simulink model "FullCarModel"  (R2023a)
settings: Solver=FixedStepAuto  StartTime=0.0  StopTime=10.0  FixedStep=5e-3  RelTol=1e-3
values from neighbouring files (symbols this model uses):
  z_r_type = 1    [FullCarParameters.m]
undefined symbols (not defined in the file or in its folder): a1F, a2F, aero, BF, CF, chassis, constants, EF, suspension
libraries: simulink x3
settings Model: Creator=Cassio de Freitas  LastModifiedBy=Cassio de Freitas
settings DataIOCC: ReturnWorkspaceOutputsName=simout

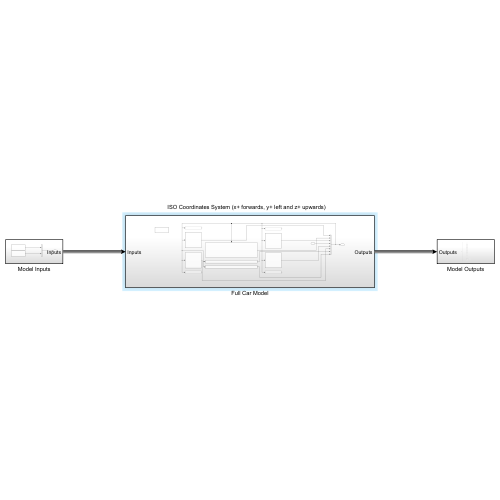
[thumbnail: Simulink's stored preview of the top-level diagram]
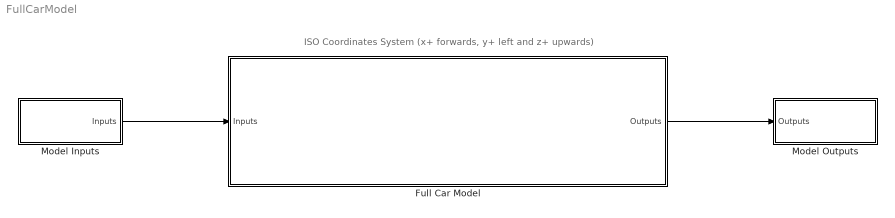
== system FullCarModel ==
  note: ISO Coordinates System (x+ forwards, y+ left and z+ upwards)
  Full Car Model : Subsystem
  Model Inputs : Subsystem
  Model Outputs : Subsystem
  wires:
  Full Car Model/1(Outputs) -> Model Outputs/1(Outputs)
  Model Inputs/1(Inputs) -> Full Car Model/1(Inputs)

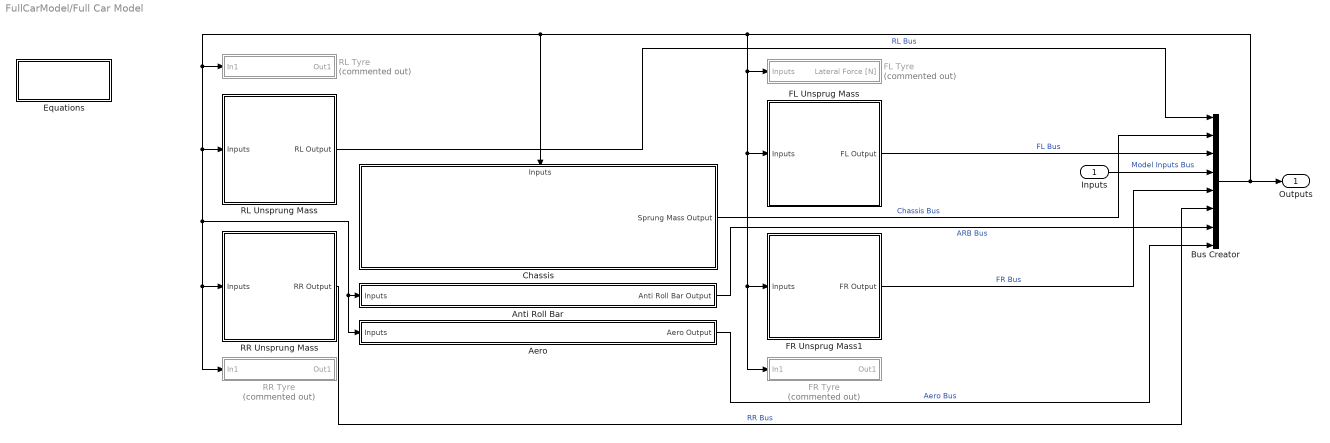
== system FullCarModel/Full Car Model ==
  Inputs : Inport
  Aero : Subsystem
  Anti Roll Bar : Subsystem
  Bus Creator : BusCreator  Inputs=8
  Chassis : Subsystem
      settings: PortSchema="{\"entries\":[{\"content\":{\"sides\":[{\"content\":{},\"type\":\"ConnectorPlacement.EquallySpacedRectSide\",\"uuid\":\"63b5c35c-1345-4ade-85d7-a7aac4cc3700\"},{\"content\":{\"connectorIds\":[\"Out1\"],\"side\":\"RIGHT\"},\"type\":\"ConnectorPlacement.EquallySpacedRectSide\",\"uuid\":\"42c6bf5f-ecea-40ec-868a-6613098306c6\"},{\"content\":{\"connectorIds\":[\"In1\"],\"side\":\"TOP\"},\"type\":\"ConnectorPlacement.EquallySpacedRectSide\",\"uuid\":\"4661345b-8a90-4c28-8ce6-d1521a801330\"}]},\"type\":\"ConnectorPlacement.EquallySpacedConnector\",\"uuid\":\"31a4e6e8-77fc-45d3-842e-fbcb04573c93\"}],\"packageUris\":[\"http://schema.mathworks.com/mf0/Connector/R2020b\"],\"version\":\"1.0\"}"
  Equations : Subsystem
  FL Tyre : Subsystem  Commented=on
  FL Unsprug Mass : Subsystem
  FR Tyre : Subsystem  Commented=on
  FR Unsprug Mass1 : Subsystem
  RL Tyre : Subsystem  Commented=on
  RL Unsprung Mass : Subsystem
  RR Tyre : Subsystem  Commented=on
  RR Unsprung Mass : Subsystem
  Outputs : Outport
  wires:
  RL Unsprung Mass/1(RL Output) -> Bus Creator/1  "RL Bus"
  Chassis/1(Sprung Mass Output) -> Bus Creator/2  "Chassis Bus"
  FL Unsprug Mass/1(FL Output) -> Bus Creator/3  "FL Bus"
  Bus Creator/1 -> Chassis/1(Inputs), RL Tyre/1(In1), RL Unsprung Mass/1(Inputs), RR Unsprung Mass/1(Inputs), RR Tyre/1(In1), Aero/1(Inputs), Anti Roll Bar/1(Inputs), FL Tyre/1(Inputs), FL Unsprug Mass/1(Inputs), FR Unsprug Mass1/1(Inputs), FR Tyre/1(In1), Outputs/1
  Inputs/1 -> Bus Creator/4  "Model Inputs Bus"
  FR Unsprug Mass1/1(FR Output) -> Bus Creator/5  "FR Bus"
  RR Unsprung Mass/1(RR Output) -> Bus Creator/6  "RR Bus"
  Anti Roll Bar/1(Anti Roll Bar Output) -> Bus Creator/7  "ARB Bus"
  Aero/1(Aero Output) -> Bus Creator/8  "Aero Bus"

== system FullCarModel/Model Inputs ==
  Driver Inputs : Subsystem
  Model Inputs Bus : BusCreator  Inputs=2
  Subsystem : Subsystem
  Inputs : Outport
  wires:
  Subsystem/1(Surface Model) -> Model Inputs Bus/1  "Surface Inputs"
  Model Inputs Bus/1 -> Inputs/1
  Driver Inputs/1(Driver Model) -> Model Inputs Bus/2  "Driver Inputs"

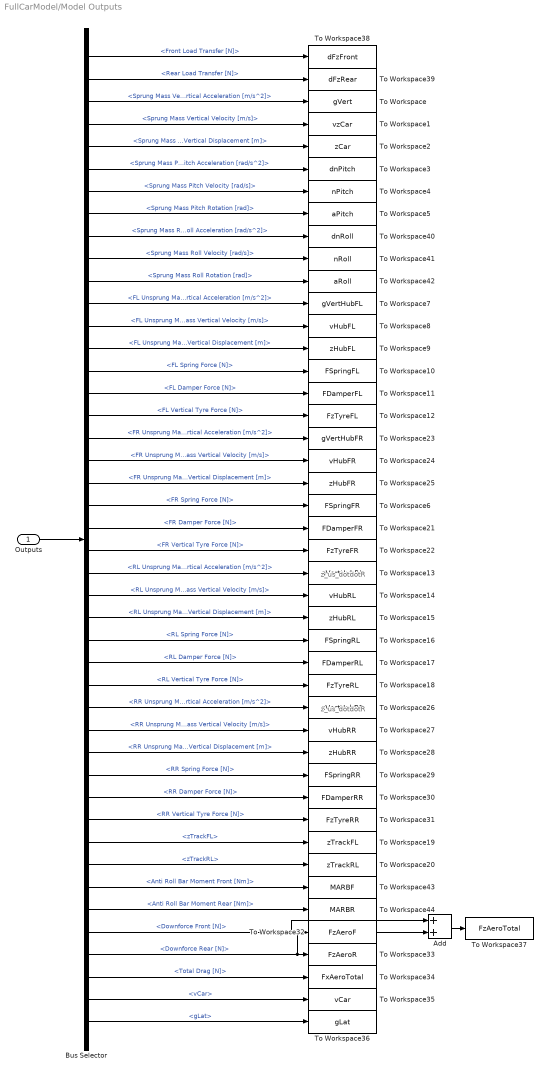
== system FullCarModel/Model Outputs ==
  note: z_us_dotdotR
  note: z_us_dotdotR
  Outputs : Inport
  Add : Sum
  Bus Selector : BusSelector  OutputSignals=FL Bus.Front Load Transfer [N],RL Bus.Rear Load Transfer [N],Chassis Bus.Sprung Mass Vertical Acceleration [m/s^2],Chassis Bus.Sprung Mass Vertical Velocity [m/s],Chassis Bus.Sprung Mass Vertical Displacement [m],Chassis Bus.Sprung Mass Pitch Acceleration [rad/s^2],Chassis Bus.Sprung Mass Pitch Velocity [rad/s],Chassis Bus.Sprung Mass Pitch Rotation [rad],Chassis Bus.Sprung Mass Roll Acceleration [rad/s^2],Chassis Bus.Sprung Mass Roll Velocity [rad/s],Chassis Bus.Sprung Mass Roll Rotation [rad],FL Bus.FL Unsprung Mass Vertical Acceleration [m/s^2],FL Bus.FL Unsprung Mass Vertical Velocity [m/s],FL Bus.FL Unsprung Mass Vertical Displacement [m],FL Bus.FL Spring Force [N],FL Bus.FL Damper Force [N],FL Bus.FL Vertical Tyre Force [N],FR Bus.FR Unsprung Mass Vertical Acceleration [m/s^2],FR Bus.FR Unsprung Mass Vertical Velocity [m/s],FR Bus.FR Unsprung Mass Vertical Displacement [m],FR Bus.FR Spring Force [N],FR Bus.FR Damper Force [N],FR Bus.FR Vertical Tyre Force [N],RL Bus.RL Unsprung Mass Vertical Acceleration [m/s^2],RL Bus.RL Unsprung Mass Vertical Velocity [m/s],RL Bus.RL Unsprung Mass Vertical Displacement [m],RL Bus.RL Spring Force [N],RL Bus.RL Damper Force [N],RL Bus.RL Vertical Tyre Force [N],RR Bus.RR Unsprung Mass Vertical Acceleration [m/s^2],RR Bus.RR Unsprung Mass Vertical Velocity [m/s],RR Bus.RR Unsprung Mass Vertical Displacement [m],RR Bus.RR Spring Force [N],RR Bus.RR Damper Force [N],RR Bus.RR Vertical Tyre Force [N],Model Inputs Bus.Surface Inputs.zTrackFL,Model Inputs Bus.Surface Inputs.zTrackRL,ARB Bus.Anti Roll Bar Moment Front [Nm],ARB Bus.Anti Roll Bar Moment Rear [Nm],Aero Bus.Downforce Front [N],Aero Bus.Downforce Rear [N],Aero Bus.Total Drag [N],Model Inputs Bus.Driver Inputs.vCar,Model Inputs Bus.Driver Inputs.gLat
  To Workspace : ToWorkspace  VariableName=gVert  SaveFormat=Timeseries  SampleTime=-1
  To Workspace1 : ToWorkspace  VariableName=vzCar  SaveFormat=Timeseries  SampleTime=-1
  To Workspace10 : ToWorkspace  VariableName=FSpringFL  SaveFormat=Timeseries  SampleTime=-1
  To Workspace11 : ToWorkspace  VariableName=FDamperFL  SaveFormat=Timeseries  SampleTime=-1
  To Workspace12 : ToWorkspace  VariableName=FzTyreFL  SaveFormat=Timeseries  SampleTime=-1
  To Workspace13 : ToWorkspace  VariableName=gVertHubRL  SaveFormat=Timeseries  SampleTime=-1
  To Workspace14 : ToWorkspace  VariableName=vHubRL  SaveFormat=Timeseries  SampleTime=-1
  To Workspace15 : ToWorkspace  VariableName=zHubRL  SaveFormat=Timeseries  SampleTime=-1
  To Workspace16 : ToWorkspace  VariableName=FSpringRL  SaveFormat=Timeseries  SampleTime=-1
  To Workspace17 : ToWorkspace  VariableName=FDamperRL  SaveFormat=Timeseries  SampleTime=-1
  To Workspace18 : ToWorkspace  VariableName=FzTyreRL  SaveFormat=Timeseries  SampleTime=-1
  To Workspace19 : ToWorkspace  VariableName=zTrackFL  SaveFormat=Timeseries  SampleTime=-1
  To Workspace2 : ToWorkspace  VariableName=zCar  SaveFormat=Timeseries  SampleTime=-1
  To Workspace20 : ToWorkspace  VariableName=zTrackRL  SaveFormat=Timeseries  SampleTime=-1
  To Workspace21 : ToWorkspace  VariableName=FDamperFR  SaveFormat=Timeseries  SampleTime=-1
  To Workspace22 : ToWorkspace  VariableName=FzTyreFR  SaveFormat=Timeseries  SampleTime=-1
  To Workspace23 : ToWorkspace  VariableName=gVertHubFR  SaveFormat=Timeseries  SampleTime=-1
  To Workspace24 : ToWorkspace  VariableName=vHubFR  SaveFormat=Timeseries  SampleTime=-1
  To Workspace25 : ToWorkspace  VariableName=zHubFR  SaveFormat=Timeseries  SampleTime=-1
  To Workspace26 : ToWorkspace  VariableName=gVertHubRR  SaveFormat=Timeseries  SampleTime=-1
  To Workspace27 : ToWorkspace  VariableName=vHubRR  SaveFormat=Timeseries  SampleTime=-1
  To Workspace28 : ToWorkspace  VariableName=zHubRR  SaveFormat=Timeseries  SampleTime=-1
  To Workspace29 : ToWorkspace  VariableName=FSpringRR  SaveFormat=Timeseries  SampleTime=-1
  To Workspace3 : ToWorkspace  VariableName=dnPitch  SaveFormat=Timeseries  SampleTime=-1
  To Workspace30 : ToWorkspace  VariableName=FDamperRR  SaveFormat=Timeseries  SampleTime=-1
  To Workspace31 : ToWorkspace  VariableName=FzTyreRR  SaveFormat=Timeseries  SampleTime=-1
  To Workspace32 : ToWorkspace  VariableName=FzAeroF  SaveFormat=Timeseries  SampleTime=-1
  To Workspace33 : ToWorkspace  VariableName=FzAeroR  SaveFormat=Timeseries  SampleTime=-1
  To Workspace34 : ToWorkspace  VariableName=FxAeroTotal  SaveFormat=Timeseries  SampleTime=-1
  To Workspace35 : ToWorkspace  VariableName=vCar  SaveFormat=Timeseries  SampleTime=-1
  To Workspace36 : ToWorkspace  VariableName=gLat  SaveFormat=Timeseries  SampleTime=-1
  To Workspace37 : ToWorkspace  VariableName=FzAeroTotal  SaveFormat=Timeseries  SampleTime=-1
  To Workspace38 : ToWorkspace  VariableName=dFzFront  SaveFormat=Timeseries  SampleTime=-1
  To Workspace39 : ToWorkspace  VariableName=dFzRear  SaveFormat=Timeseries  SampleTime=-1
  To Workspace4 : ToWorkspace  VariableName=nPitch  SaveFormat=Timeseries  SampleTime=-1
  To Workspace40 : ToWorkspace  VariableName=dnRoll  SaveFormat=Timeseries  SampleTime=-1
  To Workspace41 : ToWorkspace  VariableName=nRoll  SaveFormat=Timeseries  SampleTime=-1
  To Workspace42 : ToWorkspace  VariableName=aRoll  SaveFormat=Timeseries  SampleTime=-1
  To Workspace43 : ToWorkspace  VariableName=MARBF  SaveFormat=Timeseries  SampleTime=-1
  To Workspace44 : ToWorkspace  VariableName=MARBR  SaveFormat=Timeseries  SampleTime=-1
  To Workspace5 : ToWorkspace  VariableName=aPitch  SaveFormat=Timeseries  SampleTime=-1
  To Workspace6 : ToWorkspace  VariableName=FSpringFR  SaveFormat=Timeseries  SampleTime=-1
  To Workspace7 : ToWorkspace  VariableName=gVertHubFL  SaveFormat=Timeseries  SampleTime=-1
  To Workspace8 : ToWorkspace  VariableName=vHubFL  SaveFormat=Timeseries  SampleTime=-1
  To Workspace9 : ToWorkspace  VariableName=zHubFL  SaveFormat=Timeseries  SampleTime=-1
  wires:
  Outputs/1 -> Bus Selector/1
  Bus Selector/3 -> To Workspace/1  "<Sprung Mass Vertical Acceleration [m/s^2]>"
  Bus Selector/4 -> To Workspace1/1  "<Sprung Mass Vertical Velocity [m/s]>"
  Bus Selector/5 -> To Workspace2/1  "<Sprung Mass Vertical Displacement [m]>"
  Bus Selector/6 -> To Workspace3/1  "<Sprung Mass Pitch Acceleration [rad/s^2]>"
  Bus Selector/7 -> To Workspace4/1  "<Sprung Mass Pitch Velocity [rad/s]>"
  Bus Selector/8 -> To Workspace5/1  "<Sprung Mass Pitch Rotation [rad]>"
  Bus Selector/12 -> To Workspace7/1  "<FL Unsprung Mass Vertical Acceleration [m/s^2]>"
  Bus Selector/13 -> To Workspace8/1  "<FL Unsprung Mass Vertical Velocity [m/s]>"
  Bus Selector/14 -> To Workspace9/1  "<FL Unsprung Mass Vertical Displacement [m]>"
  Bus Selector/15 -> To Workspace10/1  "<FL Spring Force [N]>"
  Bus Selector/16 -> To Workspace11/1  "<FL Damper Force [N]>"
  Bus Selector/17 -> To Workspace12/1  "<FL Vertical Tyre Force [N]>"
  Bus Selector/24 -> To Workspace13/1  "<RL Unsprung Mass Vertical Acceleration [m/s^2]>"
  Bus Selector/25 -> To Workspace14/1  "<RL Unsprung Mass Vertical Velocity [m/s]>"
  Bus Selector/26 -> To Workspace15/1  "<RL Unsprung Mass Vertical Displacement [m]>"
  Bus Selector/27 -> To Workspace16/1  "<RL Spring Force [N]>"
  Bus Selector/28 -> To Workspace17/1  "<RL Damper Force [N]>"
  Bus Selector/29 -> To Workspace18/1  "<RL Vertical Tyre Force [N]>"
  Bus Selector/36 -> To Workspace19/1  "<zTrackFL>"
  Bus Selector/37 -> To Workspace20/1  "<zTrackRL>"
  Bus Selector/11 -> To Workspace42/1  "<Sprung Mass Roll Rotation [rad]>"
  Bus Selector/10 -> To Workspace41/1  "<Sprung Mass Roll Velocity [rad/s]>"
  Bus Selector/9 -> To Workspace40/1  "<Sprung Mass Roll Acceleration [rad/s^2]>"
  Bus Selector/38 -> To Workspace43/1  "<Anti Roll Bar Moment Front [Nm]>"
  Bus Selector/39 -> To Workspace44/1  "<Anti Roll Bar Moment Rear [Nm]>"
  Bus Selector/23 -> To Workspace22/1  "<FR Vertical Tyre Force [N]>"
  Bus Selector/22 -> To Workspace21/1  "<FR Damper Force [N]>"
  Bus Selector/21 -> To Workspace6/1  "<FR Spring Force [N]>"
  Bus Selector/20 -> To Workspace25/1  "<FR Unsprung Mass Vertical Displacement [m]>"
  Bus Selector/19 -> To Workspace24/1  "<FR Unsprung Mass Vertical Velocity [m/s]>"
  Bus Selector/18 -> To Workspace23/1  "<FR Unsprung Mass Vertical Acceleration [m/s^2]>"
  Bus Selector/35 -> To Workspace31/1  "<RR Vertical Tyre Force [N]>"
  Bus Selector/34 -> To Workspace30/1  "<RR Damper Force [N]>"
  Bus Selector/33 -> To Workspace29/1  "<RR Spring Force [N]>"
  Bus Selector/32 -> To Workspace28/1  "<RR Unsprung Mass Vertical Displacement [m]>"
  Bus Selector/31 -> To Workspace27/1  "<RR Unsprung Mass Vertical Velocity [m/s]>"
  Bus Selector/30 -> To Workspace26/1  "<RR Unsprung Mass Vertical Acceleration [m/s^2]>"
  Bus Selector/40 -> To Workspace32/1, Add/1  "<Downforce Front [N]>"
  Bus Selector/41 -> Add/2, To Workspace33/1  "<Downforce Rear [N]>"
  Bus Selector/42 -> To Workspace34/1  "<Total Drag [N]>"
  Bus Selector/43 -> To Workspace35/1  "<vCar>"
  Bus Selector/44 -> To Workspace36/1  "<gLat>"
  Add/1 -> To Workspace37/1
  Bus Selector/2 -> To Workspace39/1  "<Rear Load Transfer [N]>"
  Bus Selector/1 -> To Workspace38/1  "<Front Load Transfer [N]>"

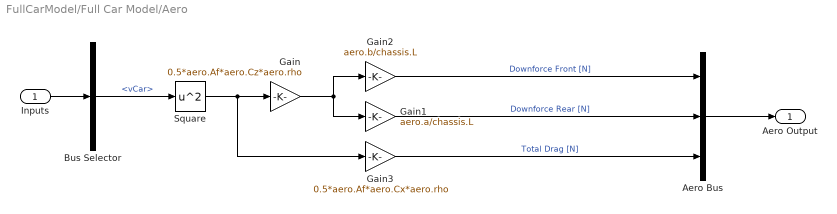
== system FullCarModel/Full Car Model/Aero ==
  Inputs : Inport
  Aero Bus : BusCreator  Inputs=3
  Bus Selector : BusSelector  OutputSignals=Model Inputs Bus.Driver Inputs.vCar
  Gain : Gain  Gain=0.5*aero.Af*aero.Cz*aero.rho
  Gain1 : Gain  Gain=aero.a/chassis.L
  Gain2 : Gain  Gain=aero.b/chassis.L
  Gain3 : Gain  Gain=0.5*aero.Af*aero.Cx*aero.rho
  Square : Math  Operator=square
  Aero Output : Outport
  wires:
  Aero Bus/1 -> Aero Output/1
  Inputs/1 -> Bus Selector/1
  Bus Selector/1 -> Square/1  "<vCar>"
  Square/1 -> Gain3/1, Gain/1
  Gain/1 -> Gain1/1, Gain2/1
  Gain2/1 -> Aero Bus/1  "Downforce Front [N]"
  Gain1/1 -> Aero Bus/2  "Downforce Rear [N]"
  Gain3/1 -> Aero Bus/3  "Total Drag [N]"

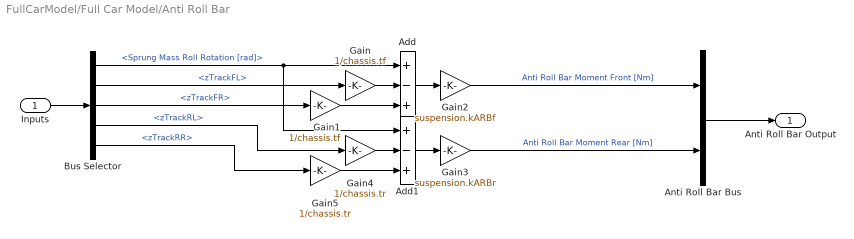
== system FullCarModel/Full Car Model/Anti Roll Bar ==
  Inputs : Inport
  Add : Sum  Inputs=+-+
  Add1 : Sum  Inputs=+-+
  Anti Roll Bar Bus : BusCreator  Inputs=2
  Bus Selector : BusSelector  OutputSignals=Chassis Bus.Sprung Mass Roll Rotation [rad],Model Inputs Bus.Surface Inputs.zTrackFL,Model Inputs Bus.Surface Inputs.zTrackFR,Model Inputs Bus.Surface Inputs.zTrackRL,Model Inputs Bus.Surface Inputs.zTrackRR
  Gain : Gain  Gain=1/chassis.tf
  Gain1 : Gain  Gain=1/chassis.tf
  Gain2 : Gain  Gain=suspension.kARBf
  Gain3 : Gain  Gain=suspension.kARBr
  Gain4 : Gain  Gain=1/chassis.tr
  Gain5 : Gain  Gain=1/chassis.tr
  Anti Roll Bar Output : Outport
  wires:
  Inputs/1 -> Bus Selector/1
  Bus Selector/1 -> Add1/1, Add/1  "<Sprung Mass Roll Rotation [rad]>"
  Bus Selector/2 -> Gain/1  "<zTrackFL>"
  Bus Selector/3 -> Gain1/1  "<zTrackFR>"
  Gain2/1 -> Anti Roll Bar Bus/1  "Anti Roll Bar Moment Front [Nm]"
  Gain3/1 -> Anti Roll Bar Bus/2  "Anti Roll Bar Moment Rear [Nm]"
  Gain/1 -> Add/2
  Gain1/1 -> Add/3
  Add/1 -> Gain2/1
  Add1/1 -> Gain3/1
  Bus Selector/4 -> Gain4/1  "<zTrackRL>"
  Bus Selector/5 -> Gain5/1  "<zTrackRR>"
  Gain4/1 -> Add1/2
  Gain5/1 -> Add1/3
  Anti Roll Bar Bus/1 -> Anti Roll Bar Output/1

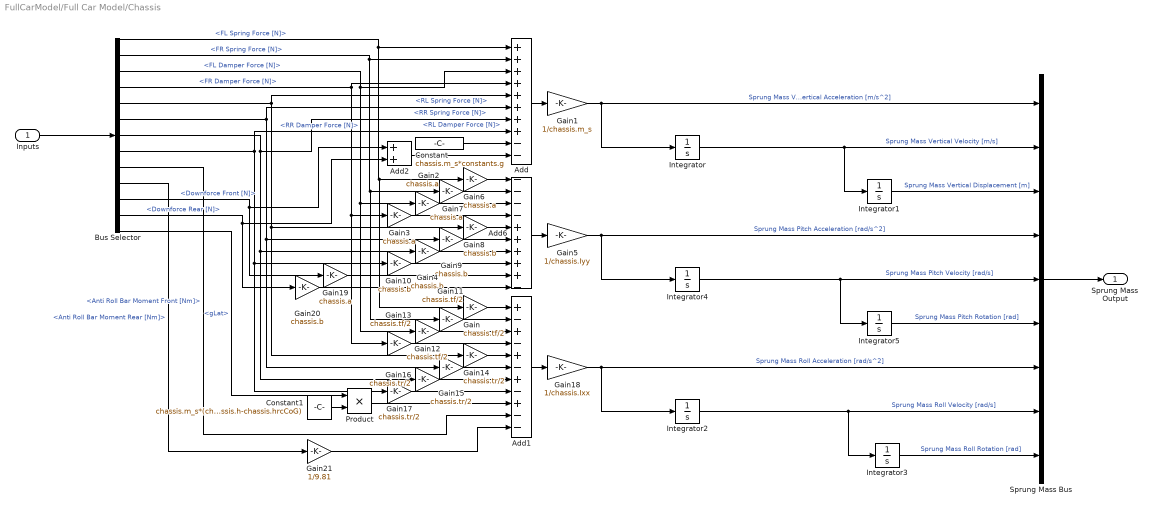
== system FullCarModel/Full Car Model/Chassis ==
  Inputs : Inport
  Add : Sum  Inputs=++++++++--
  Add1 : Sum  Inputs=+-+-+-+-+--
  Add2 : Sum
  Add6 : Sum  Inputs=----+++++-
  Bus Selector : BusSelector  OutputSignals=FL Bus.FL Spring Force [N],FR Bus.FR Spring Force [N],FL Bus.FL Damper Force [N],FR Bus.FR Damper Force [N],RL Bus.RL Spring Force [N],RR Bus.RR Spring Force [N],RL Bus.RL Damper Force [N],RR Bus.RR Damper Force [N],ARB Bus.Anti Roll Bar Moment Front [Nm],ARB Bus.Anti Roll Bar Moment Rear [Nm],Aero Bus.Downforce Front [N],Aero Bus.Downforce Rear [N],Model Inputs Bus.Driver Inputs.gLat
  Constant : Constant  Value=chassis.m_s*constants.g
  Constant1 : Constant  Value=chassis.m_s*(chassis.h-chassis.hrcCoG)
  Gain{,11..13} (4 alike) : Gain  Gain=chassis.tf/2
  Gain1 : Gain  Gain=1/chassis.m_s
  Gain{4,8..10,20} (5 alike) : Gain  Gain=chassis.b
  Gain{14..17} (4 alike) : Gain  Gain=chassis.tr/2
  Gain18 : Gain  Gain=1/chassis.Ixx
  Gain{2..3,6..7,19} (5 alike) : Gain  Gain=chassis.a
  Gain21 : Gain  Gain=1/9.81
  Gain5 : Gain  Gain=1/chassis.Iyy
  Integrator{,1..5} (6 alike) : Integrator
  Product : Product
  Sprung Mass Bus : BusCreator  Inputs=9
  Sprung Mass Output : Outport
  wires:
  Integrator4/1 -> Integrator5/1, Sprung Mass Bus/5  "Sprung Mass Pitch Velocity [rad/s]"
  Gain5/1 -> Integrator4/1, Sprung Mass Bus/4  "Sprung Mass Pitch Acceleration [rad/s^2]"
  Gain1/1 -> Integrator/1, Sprung Mass Bus/1  "Sprung Mass Vertical Acceleration [m/s^2]"
  Integrator1/1 -> Sprung Mass Bus/3  "Sprung Mass Vertical Displacement [m]"
  Add/1 -> Gain1/1
  Add6/1 -> Gain5/1
  Integrator5/1 -> Sprung Mass Bus/6  "Sprung Mass Pitch Rotation [rad]"
  Integrator/1 -> Integrator1/1, Sprung Mass Bus/2  "Sprung Mass Vertical Velocity [m/s]"
  Sprung Mass Bus/1 -> Sprung Mass Output/1
  Inputs/1 -> Bus Selector/1
  Constant/1 -> Add/9
  Bus Selector/1 -> Gain/1, Gain6/1, Add/1  "<FL Spring Force [N]>"
  Bus Selector/2 -> Gain11/1, Gain7/1, Add/2  "<FR Spring Force [N]>"
  Bus Selector/3 -> Gain12/1, Gain2/1, Add/3  "<FL Damper Force [N]>"
  Bus Selector/4 -> Gain13/1, Gain3/1, Add/4  "<FR Damper Force [N]>"
  Bus Selector/5 -> Gain14/1, Gain8/1, Add/5  "<RL Spring Force [N]>"
  Bus Selector/6 -> Gain15/1, Gain9/1, Add/6  "<RR Spring Force [N]>"
  Bus Selector/7 -> Gain16/1, Gain4/1, Add/7  "<RL Damper Force [N]>"
  Bus Selector/8 -> Gain17/1, Gain10/1, Add/8  "<RR Damper Force [N]>"
  Gain6/1 -> Add6/1
  Gain7/1 -> Add6/2
  Gain2/1 -> Add6/3
  Gain3/1 -> Add6/4
  Gain8/1 -> Add6/5
  Gain9/1 -> Add6/6
  Gain4/1 -> Add6/7
  Gain10/1 -> Add6/8
  Gain/1 -> Add1/1
  Gain11/1 -> Add1/2
  Gain12/1 -> Add1/3
  Gain13/1 -> Add1/4
  Gain14/1 -> Add1/5
  Gain15/1 -> Add1/6
  Gain16/1 -> Add1/7
  Gain17/1 -> Add1/8
  Bus Selector/9 -> Add1/10  "<Anti Roll Bar Moment Front [Nm]>"
  Bus Selector/10 -> Gain21/1  "<Anti Roll Bar Moment Rear [Nm]>"
  Add1/1 -> Gain18/1
  Gain18/1 -> Sprung Mass Bus/7, Integrator2/1  "Sprung Mass Roll Acceleration [rad/s^2]"
  Integrator2/1 -> Integrator3/1, Sprung Mass Bus/8  "Sprung Mass Roll Velocity [rad/s]"
  Integrator3/1 -> Sprung Mass Bus/9  "Sprung Mass Roll Rotation [rad]"
  Bus Selector/11 -> Gain19/1, Add2/1  "<Downforce Front [N]>"
  Bus Selector/12 -> Gain20/1, Add2/2  "<Downforce Rear [N]>"
  Add2/1 -> Add/10
  Gain19/1 -> Add6/9
  Gain20/1 -> Add6/10
  Product/1 -> Add1/9
  Constant1/1 -> Product/2
  Bus Selector/13 -> Product/1  "<gLat>"
  Gain21/1 -> Add1/11

== system FullCarModel/Full Car Model/Equations ==

== system FullCarModel/Full Car Model/FL Tyre ==
  Inputs : Inport
  Bus Selector : BusSelector  OutputSignals=signal1,signal2
  Pacejka FL Lateral Tyre Model : Subsystem
  Lateral Force [N] : Outport
  wires:
  Pacejka FL Lateral Tyre Model/1(Lateral Force [N]) -> Lateral Force [N]/1
  Inputs/1 -> Bus Selector/1

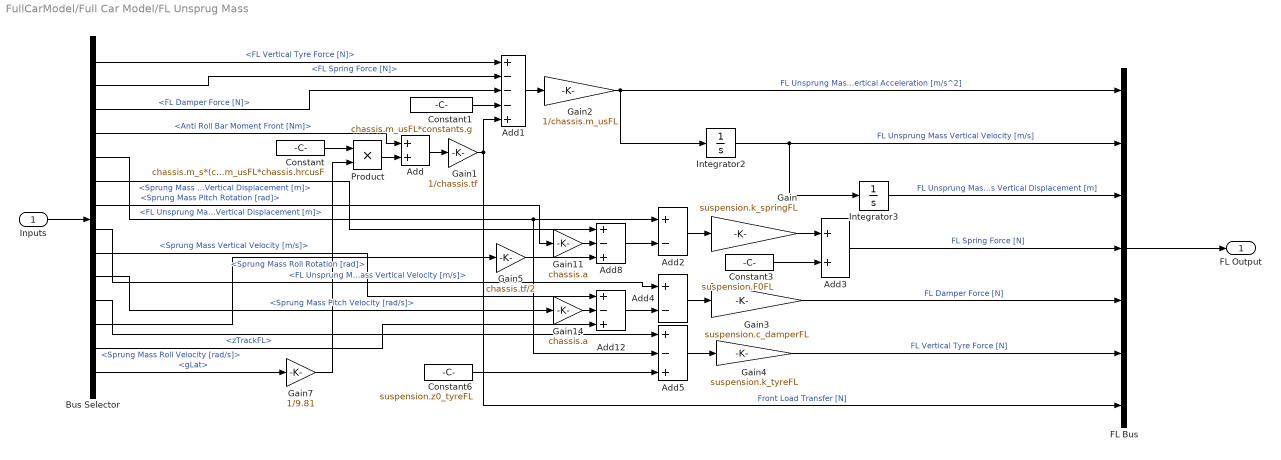
== system FullCarModel/Full Car Model/FL Unsprug Mass ==
  Inputs : Inport
  Add : Sum
  Add1 : Sum  Inputs=+---+
  Add12 : Sum  Inputs=+-+
  Add2 : Sum  Inputs=+-
  Add3 : Sum
  Add4 : Sum  Inputs=+-
  Add5 : Sum  Inputs=+-+
  Add8 : Sum  Inputs=+-+
  Bus Selector : BusSelector  OutputSignals=FL Bus.FL Vertical Tyre Force [N],FL Bus.FL Spring Force [N],FL Bus.FL Damper Force [N],ARB Bus.Anti Roll Bar Moment Front [Nm],FL Bus.FL Unsprung Mass Vertical Displacement [m],Chassis Bus.Sprung Mass Vertical Displacement [m],Chassis Bus.Sprung Mass Pitch Rotation [rad],FL Bus.FL Unsprung Mass Vertical Velocity [m/s],Chassis Bus.Sprung Mass Vertical Velocity [m/s],Chassis Bus.Sprung Mass Pitch Velocity [rad/s],Model Inputs Bus.Surface Inputs.zTrackFL,Chassis Bus.Sprung Mass Roll Rotation [rad],Chassis Bus.Sprung Mass Roll Velocity [rad/s],Model Inputs Bus.Driver Inputs.gLat
  Constant : Constant  Value=chassis.m_s*(chassis.b/chassis.L)*chassis.hrcF+2*chassis.m_usFL*chassis.hrcusF
  Constant1 : Constant  Value=chassis.m_usFL*constants.g
  Constant3 : Constant  Value=suspension.F0FL
  Constant6 : Constant  Value=suspension.z0_tyreFL
  FL Bus : BusCreator  Inputs=7
  Gain : Gain  Gain=suspension.k_springFL
  Gain1 : Gain  Gain=1/chassis.tf
  Gain11 : Gain  Gain=chassis.a
  Gain14 : Gain  Gain=chassis.a
  Gain2 : Gain  Gain=1/chassis.m_usFL
  Gain3 : Gain  Gain=suspension.c_damperFL
  Gain4 : Gain  Gain=suspension.k_tyreFL
  Gain5 : Gain  Gain=chassis.tf/2
  Gain7 : Gain  Gain=1/9.81
  Integrator2 : Integrator
  Integrator3 : Integrator
  Product : Product
  FL Output : Outport
  wires:
  Integrator3/1 -> FL Bus/3  "FL Unsprung Mass Vertical Displacement [m]"
  Add1/1 -> Gain2/1
  Integrator2/1 -> FL Bus/2, Integrator3/1  "FL Unsprung Mass Vertical Velocity [m/s]"
  Gain2/1 -> Integrator2/1, FL Bus/1  "FL Unsprung Mass Vertical Acceleration [m/s^2]"
  Gain11/1 -> Add8/2
  Bus Selector/6 -> Add8/1  "<Sprung Mass Vertical Displacement [m]>"
  Add8/1 -> Add2/2
  Add3/1 -> FL Bus/4  "FL Spring Force [N]"
  Gain/1 -> Add3/1
  Add4/1 -> Gain3/1
  Constant3/1 -> Add3/2
  Bus Selector/5 -> Add2/1, Add5/2  "<FL Unsprung Mass Vertical Displacement [m]>"
  Gain3/1 -> FL Bus/5  "FL Damper Force [N]"
  Gain14/1 -> Add12/2
  Add2/1 -> Gain/1
  Add12/1 -> Add4/2
  Add5/1 -> Gain4/1
  Constant6/1 -> Add5/3
  Gain4/1 -> FL Bus/6  "FL Vertical Tyre Force [N]"
  Bus Selector/3 -> Add1/3  "<FL Damper Force [N]>"
  Bus Selector/1 -> Add1/1  "<FL Vertical Tyre Force [N]>"
  Constant1/1 -> Add1/4
  Bus Selector/8 -> Add4/1  "<FL Unsprung Mass Vertical Velocity [m/s]>"
  Bus Selector/10 -> Gain14/1  "<Sprung Mass Pitch Velocity [rad/s]>"
  FL Bus/1 -> FL Output/1
  Inputs/1 -> Bus Selector/1
  Bus Selector/2 -> Add1/2  "<FL Spring Force [N]>"
  Bus Selector/7 -> Gain11/1  "<Sprung Mass Pitch Rotation [rad]>"
  Bus Selector/9 -> Add12/1  "<Sprung Mass Vertical Velocity [m/s]>"
  Bus Selector/11 -> Add5/1  "<zTrackFL>"
  Bus Selector/4 -> Add/1  "<Anti Roll Bar Moment Front [Nm]>"
  Add/1 -> Gain1/1
  Bus Selector/12 -> Gain5/1  "<Sprung Mass Roll Rotation [rad]>"
  Gain5/1 -> Add8/3
  Bus Selector/13 -> Add12/3  "<Sprung Mass Roll Velocity [rad/s]>"
  Product/1 -> Add/2
  Constant/1 -> Product/1
  Bus Selector/14 -> Gain7/1  "<gLat>"
  Gain1/1 -> FL Bus/7, Add1/5  "Front Load Transfer [N]"
  Gain7/1 -> Product/2

== system FullCarModel/Full Car Model/FR Tyre ==
  In1 : Inport
  Out1 : Outport
  wires:
  In1/1 -> Out1/1

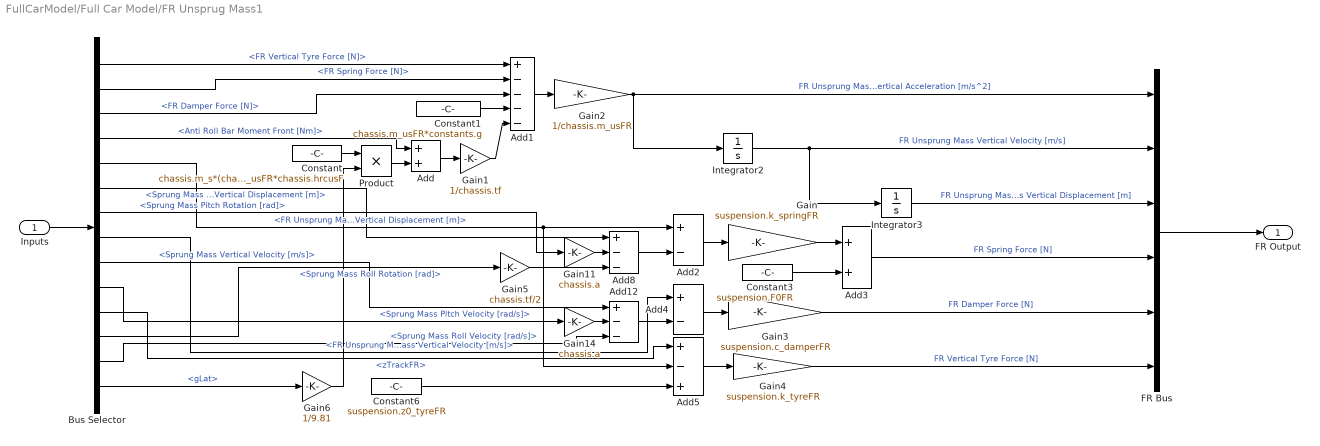
== system FullCarModel/Full Car Model/FR Unsprug Mass1 ==
  Inputs : Inport
  Add : Sum
  Add1 : Sum  Inputs=+----
  Add12 : Sum  Inputs=+--
  Add2 : Sum  Inputs=+-
  Add3 : Sum
  Add4 : Sum  Inputs=+-
  Add5 : Sum  Inputs=+-+
  Add8 : Sum  Inputs=+--
  Bus Selector : BusSelector  OutputSignals=FR Bus.FR Vertical Tyre Force [N],FR Bus.FR Spring Force [N],FR Bus.FR Damper Force [N],ARB Bus.Anti Roll Bar Moment Front [Nm],FR Bus.FR Unsprung Mass Vertical Displacement [m],Chassis Bus.Sprung Mass Vertical Displacement [m],Chassis Bus.Sprung Mass Pitch Rotation [rad],FR Bus.FR Unsprung Mass Vertical Velocity [m/s],Chassis Bus.Sprung Mass Vertical Velocity [m/s],Chassis Bus.Sprung Mass Pitch Velocity [rad/s],Model Inputs Bus.Surface Inputs.zTrackFR,Chassis Bus.Sprung Mass Roll Rotation [rad],Chassis Bus.Sprung Mass Roll Velocity [rad/s],Model Inputs Bus.Driver Inputs.gLat
  Constant : Constant  Value=chassis.m_s*(chassis.b/chassis.L)*chassis.hrcF+2*chassis.m_usFR*chassis.hrcusF
  Constant1 : Constant  Value=chassis.m_usFR*constants.g
  Constant3 : Constant  Value=suspension.F0FR
  Constant6 : Constant  Value=suspension.z0_tyreFR
  FR Bus : BusCreator  Inputs=6
  Gain : Gain  Gain=suspension.k_springFR
  Gain1 : Gain  Gain=1/chassis.tf
  Gain11 : Gain  Gain=chassis.a
  Gain14 : Gain  Gain=chassis.a
  Gain2 : Gain  Gain=1/chassis.m_usFR
  Gain3 : Gain  Gain=suspension.c_damperFR
  Gain4 : Gain  Gain=suspension.k_tyreFR
  Gain5 : Gain  Gain=chassis.tf/2
  Gain6 : Gain  Gain=1/9.81
  Integrator2 : Integrator
  Integrator3 : Integrator
  Product : Product
  FR Output : Outport
  wires:
  Bus Selector/11 -> Add5/1  "<zTrackFR>"
  Bus Selector/9 -> Add12/1  "<Sprung Mass Vertical Velocity [m/s]>"
  Bus Selector/7 -> Gain11/1  "<Sprung Mass Pitch Rotation [rad]>"
  Bus Selector/2 -> Add1/2  "<FR Spring Force [N]>"
  Inputs/1 -> Bus Selector/1
  FR Bus/1 -> FR Output/1
  Bus Selector/10 -> Gain14/1  "<Sprung Mass Pitch Velocity [rad/s]>"
  Bus Selector/8 -> Add4/1  "<FR Unsprung Mass Vertical Velocity [m/s]>"
  Constant1/1 -> Add1/4
  Bus Selector/1 -> Add1/1  "<FR Vertical Tyre Force [N]>"
  Bus Selector/3 -> Add1/3  "<FR Damper Force [N]>"
  Gain4/1 -> FR Bus/6  "FR Vertical Tyre Force [N]"
  Constant6/1 -> Add5/3
  Add5/1 -> Gain4/1
  Add12/1 -> Add4/2
  Add2/1 -> Gain/1
  Gain14/1 -> Add12/2
  Gain3/1 -> FR Bus/5  "FR Damper Force [N]"
  Bus Selector/5 -> Add2/1, Add5/2  "<FR Unsprung Mass Vertical Displacement [m]>"
  Constant3/1 -> Add3/2
  Add4/1 -> Gain3/1
  Gain/1 -> Add3/1
  Add3/1 -> FR Bus/4  "FR Spring Force [N]"
  Add8/1 -> Add2/2
  Bus Selector/6 -> Add8/1  "<Sprung Mass Vertical Displacement [m]>"
  Gain11/1 -> Add8/2
  Gain2/1 -> FR Bus/1, Integrator2/1  "FR Unsprung Mass Vertical Acceleration [m/s^2]"
  Integrator2/1 -> Integrator3/1, FR Bus/2  "FR Unsprung Mass Vertical Velocity [m/s]"
  Add1/1 -> Gain2/1
  Integrator3/1 -> FR Bus/3  "FR Unsprung Mass Vertical Displacement [m]"
  Add/1 -> Gain1/1
  Gain1/1 -> Add1/5
  Bus Selector/4 -> Add/1  "<Anti Roll Bar Moment Front [Nm]>"
  Gain5/1 -> Add8/3
  Bus Selector/12 -> Gain5/1  "<Sprung Mass Roll Rotation [rad]>"
  Bus Selector/13 -> Add12/3  "<Sprung Mass Roll Velocity [rad/s]>"
  Product/1 -> Add/2
  Constant/1 -> Product/1
  Bus Selector/14 -> Gain6/1  "<gLat>"
  Gain6/1 -> Product/2

== system FullCarModel/Full Car Model/RL Tyre ==
  In1 : Inport
  Out1 : Outport
  wires:
  In1/1 -> Out1/1

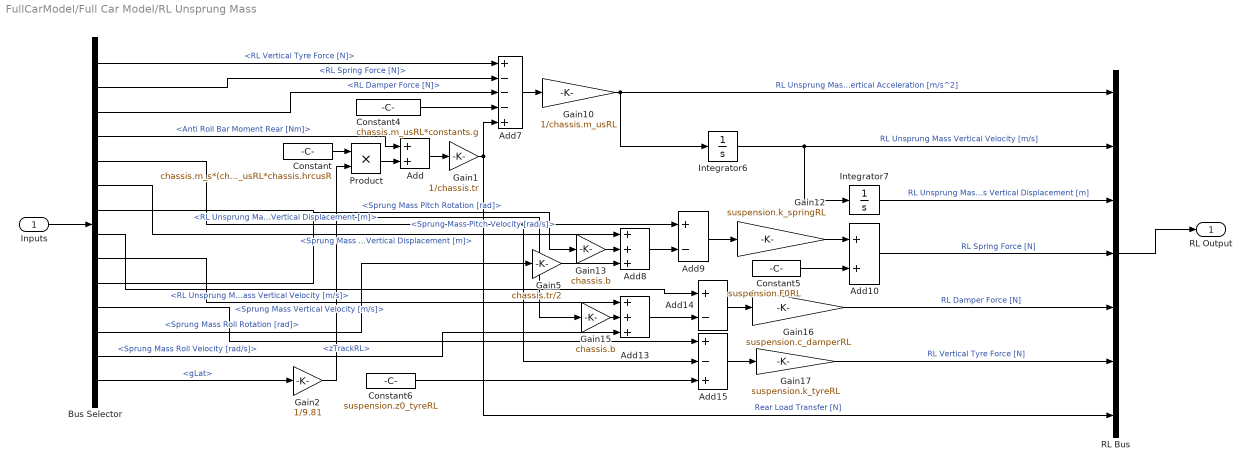
== system FullCarModel/Full Car Model/RL Unsprung Mass ==
  Inputs : Inport
  Add : Sum
  Add10 : Sum
  Add13 : Sum  Inputs=+++
  Add14 : Sum  Inputs=+-
  Add15 : Sum  Inputs=+-+
  Add7 : Sum  Inputs=+---+
  Add8 : Sum  Inputs=+++
  Add9 : Sum  Inputs=+-
  Bus Selector : BusSelector  OutputSignals=RL Bus.RL Vertical Tyre Force [N],RL Bus.RL Spring Force [N],RL Bus.RL Damper Force [N],ARB Bus.Anti Roll Bar Moment Rear [Nm],RL Bus.RL Unsprung Mass Vertical Displacement [m],Chassis Bus.Sprung Mass Vertical Displacement [m],Chassis Bus.Sprung Mass Pitch Rotation [rad],RL Bus.RL Unsprung Mass Vertical Velocity [m/s],Chassis Bus.Sprung Mass Vertical Velocity [m/s],Chassis Bus.Sprung Mass Pitch Velocity [rad/s],Model Inputs Bus.Surface Inputs.zTrackRL,Chassis Bus.Sprung Mass Roll Rotation [rad],Chassis Bus.Sprung Mass Roll Velocity [rad/s],Model Inputs Bus.Driver Inputs.gLat
  Constant : Constant  Value=chassis.m_s*(chassis.a/chassis.L)*chassis.hrcR+2*chassis.m_usRL*chassis.hrcusR
  Constant4 : Constant  Value=chassis.m_usRL*constants.g
  Constant5 : Constant  Value=suspension.F0RL
  Constant6 : Constant  Value=suspension.z0_tyreRL
  Gain1 : Gain  Gain=1/chassis.tr
  Gain10 : Gain  Gain=1/chassis.m_usRL
  Gain12 : Gain  Gain=suspension.k_springRL
  Gain13 : Gain  Gain=chassis.b
  Gain15 : Gain  Gain=chassis.b
  Gain16 : Gain  Gain=suspension.c_damperRL
  Gain17 : Gain  Gain=suspension.k_tyreRL
  Gain2 : Gain  Gain=1/9.81
  Gain5 : Gain  Gain=chassis.tr/2
  Integrator6 : Integrator
  Integrator7 : Integrator
  Product : Product
  RL Bus : BusCreator  Inputs=7
  RL Output : Outport
  wires:
  Integrator7/1 -> RL Bus/3  "RL Unsprung Mass Vertical Displacement [m]"
  Add7/1 -> Gain10/1
  Gain10/1 -> Integrator6/1, RL Bus/1  "RL Unsprung Mass Vertical Acceleration [m/s^2]"
  Integrator6/1 -> RL Bus/2, Integrator7/1  "RL Unsprung Mass Vertical Velocity [m/s]"
  Add8/1 -> Add9/2
  Add9/1 -> Gain12/1
  Gain16/1 -> RL Bus/5  "RL Damper Force [N]"
  Add13/1 -> Add14/2
  Gain13/1 -> Add8/2
  Gain12/1 -> Add10/1
  Add14/1 -> Gain16/1
  Add10/1 -> RL Bus/4  "RL Spring Force [N]"
  Gain15/1 -> Add13/2
  Constant5/1 -> Add10/2
  Gain17/1 -> RL Bus/6  "RL Vertical Tyre Force [N]"
  Add15/1 -> Gain17/1
  Bus Selector/1 -> Add7/1  "<RL Vertical Tyre Force [N]>"
  Bus Selector/3 -> Add7/3  "<RL Damper Force [N]>"
  Constant4/1 -> Add7/4
  Bus Selector/5 -> Add9/1, Add15/2  "<RL Unsprung Mass Vertical Displacement [m]>"
  Bus Selector/6 -> Add8/1  "<Sprung Mass Vertical Displacement [m]>"
  Bus Selector/7 -> Gain13/1  "<Sprung Mass Pitch Rotation [rad]>"
  Bus Selector/8 -> Add14/1  "<RL Unsprung Mass Vertical Velocity [m/s]>"
  Bus Selector/9 -> Add13/1  "<Sprung Mass Vertical Velocity [m/s]>"
  Bus Selector/10 -> Gain15/1  "<Sprung Mass Pitch Velocity [rad/s]>"
  Bus Selector/11 -> Add15/1  "<zTrackRL>"
  Constant6/1 -> Add15/3
  RL Bus/1 -> RL Output/1
  Inputs/1 -> Bus Selector/1
  Bus Selector/2 -> Add7/2  "<RL Spring Force [N]>"
  Add/1 -> Gain1/1
  Bus Selector/4 -> Add/1  "<Anti Roll Bar Moment Rear [Nm]>"
  Gain5/1 -> Add8/3
  Bus Selector/12 -> Gain5/1  "<Sprung Mass Roll Rotation [rad]>"
  Bus Selector/13 -> Add13/3  "<Sprung Mass Roll Velocity [rad/s]>"
  Product/1 -> Add/2
  Constant/1 -> Product/1
  Bus Selector/14 -> Gain2/1  "<gLat>"
  Gain1/1 -> RL Bus/7, Add7/5  "Rear Load Transfer [N]"
  Gain2/1 -> Product/2

== system FullCarModel/Full Car Model/RR Tyre ==
  In1 : Inport
  Out1 : Outport
  wires:
  In1/1 -> Out1/1

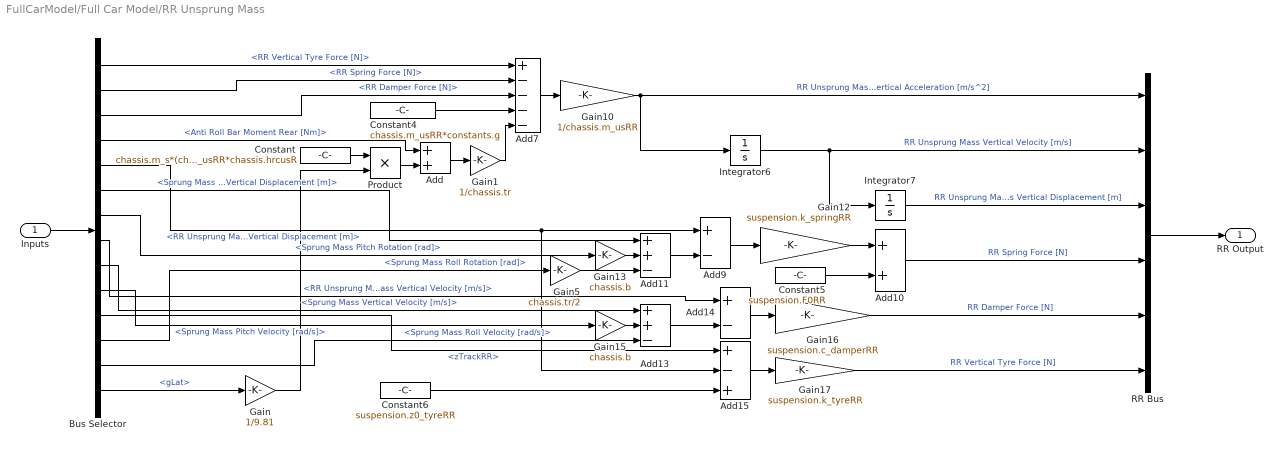
== system FullCarModel/Full Car Model/RR Unsprung Mass ==
  Inputs : Inport
  Add : Sum
  Add10 : Sum
  Add11 : Sum  Inputs=++-
  Add13 : Sum  Inputs=++-
  Add14 : Sum  Inputs=+-
  Add15 : Sum  Inputs=+-+
  Add7 : Sum  Inputs=+----
  Add9 : Sum  Inputs=+-
  Bus Selector : BusSelector  OutputSignals=RR Bus.RR Vertical Tyre Force [N],RR Bus.RR Spring Force [N],RR Bus.RR Damper Force [N],ARB Bus.Anti Roll Bar Moment Rear [Nm],RR Bus.RR Unsprung Mass Vertical Displacement [m],Chassis Bus.Sprung Mass Vertical Displacement [m],Chassis Bus.Sprung Mass Pitch Rotation [rad],RR Bus.RR Unsprung Mass Vertical Velocity [m/s],Chassis Bus.Sprung Mass Vertical Velocity [m/s],Chassis Bus.Sprung Mass Pitch Velocity [rad/s],Model Inputs Bus.Surface Inputs.zTrackRR,Chassis Bus.Sprung Mass Roll Rotation [rad],Chassis Bus.Sprung Mass Roll Velocity [rad/s],Model Inputs Bus.Driver Inputs.gLat
  Constant : Constant  Value=chassis.m_s*(chassis.a/chassis.L)*chassis.hrcR+2*chassis.m_usRR*chassis.hrcusR
  Constant4 : Constant  Value=chassis.m_usRR*constants.g
  Constant5 : Constant  Value=suspension.F0RR
  Constant6 : Constant  Value=suspension.z0_tyreRR
  Gain : Gain  Gain=1/9.81
  Gain1 : Gain  Gain=1/chassis.tr
  Gain10 : Gain  Gain=1/chassis.m_usRR
  Gain12 : Gain  Gain=suspension.k_springRR
  Gain13 : Gain  Gain=chassis.b
  Gain15 : Gain  Gain=chassis.b
  Gain16 : Gain  Gain=suspension.c_damperRR
  Gain17 : Gain  Gain=suspension.k_tyreRR
  Gain5 : Gain  Gain=chassis.tr/2
  Integrator6 : Integrator
  Integrator7 : Integrator
  Product : Product
  RR Bus : BusCreator  Inputs=6
  RR Output : Outport
  wires:
  Bus Selector/2 -> Add7/2  "<RR Spring Force [N]>"
  Inputs/1 -> Bus Selector/1
  RR Bus/1 -> RR Output/1
  Constant6/1 -> Add15/3
  Bus Selector/11 -> Add15/1  "<zTrackRR>"
  Bus Selector/10 -> Gain15/1  "<Sprung Mass Pitch Velocity [rad/s]>"
  Bus Selector/9 -> Add13/1  "<Sprung Mass Vertical Velocity [m/s]>"
  Bus Selector/8 -> Add14/1  "<RR Unsprung Mass Vertical Velocity [m/s]>"
  Bus Selector/7 -> Gain13/1  "<Sprung Mass Pitch Rotation [rad]>"
  Bus Selector/6 -> Add11/1  "<Sprung Mass Vertical Displacement [m]>"
  Bus Selector/5 -> Add15/2, Add9/1  "<RR Unsprung Mass Vertical Displacement [m]>"
  Constant4/1 -> Add7/4
  Bus Selector/3 -> Add7/3  "<RR Damper Force [N]>"
  Bus Selector/1 -> Add7/1  "<RR Vertical Tyre Force [N]>"
  Add15/1 -> Gain17/1
  Gain17/1 -> RR Bus/6  "RR Vertical Tyre Force [N]"
  Constant5/1 -> Add10/2
  Gain15/1 -> Add13/2
  Add10/1 -> RR Bus/4  "RR Spring Force [N]"
  Add14/1 -> Gain16/1
  Gain12/1 -> Add10/1
  Gain13/1 -> Add11/2
  Add13/1 -> Add14/2
  Gain16/1 -> RR Bus/5  "RR Damper Force [N]"
  Add9/1 -> Gain12/1
  Add11/1 -> Add9/2
  Integrator6/1 -> Integrator7/1, RR Bus/2  "RR Unsprung Mass Vertical Velocity [m/s]"
  Gain10/1 -> Integrator6/1, RR Bus/1  "RR Unsprung Mass Vertical Acceleration [m/s^2]"
  Add7/1 -> Gain10/1
  Integrator7/1 -> RR Bus/3  "RR Unsprung Mass Vertical Displacement [m]"
  Bus Selector/4 -> Add/1  "<Anti Roll Bar Moment Rear [Nm]>"
  Add/1 -> Gain1/1
  Gain1/1 -> Add7/5
  Gain5/1 -> Add11/3
  Bus Selector/12 -> Gain5/1  "<Sprung Mass Roll Rotation [rad]>"
  Bus Selector/13 -> Add13/3  "<Sprung Mass Roll Velocity [rad/s]>"
  Product/1 -> Add/2
  Constant/1 -> Product/1
  Bus Selector/14 -> Gain/1  "<gLat>"
  Gain/1 -> Product/2

== system FullCarModel/Model Inputs/Driver Inputs ==
  Driver Input Bus : BusCreator  Inputs=2
  Ramp : simulink/Sources/Ramp  slope=0  start=0  InitialOutput=0
  Ramp1 : simulink/Sources/Ramp  slope=0.8  start=0  InitialOutput=0
  Driver Model : Outport
  wires:
  Driver Input Bus/1 -> Driver Model/1
  Ramp/1 -> Driver Input Bus/1  "vCar"
  Ramp1/1 -> Driver Input Bus/2  "gLat"

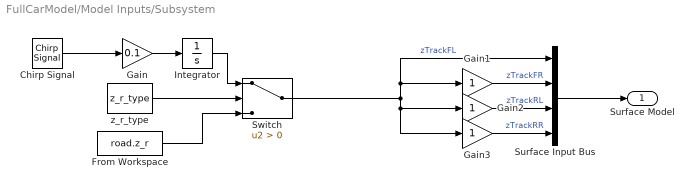
== system FullCarModel/Model Inputs/Subsystem ==
  Chirp Signal : simulink/Sources/Chirp Signal  f1=0.1  T=100  f2=50
  From Workspace : FromWorkspace  VariableName=road.z_r
  Gain : Gain  Gain=0.1
  Gain1 : Gain
  Gain2 : Gain
  Gain3 : Gain
  Integrator : Integrator
  Surface Input Bus : BusCreator  Inputs=4
  Switch : Switch  Criteria=u2 > Threshold  SaturateOnIntegerOverflow=off  InputSameDT=off
  z_r_type : Constant  Value=z_r_type
  Surface Model : Outport
  wires:
  Switch/1 -> Gain2/1, Gain3/1, Gain1/1, Surface Input Bus/1  "zTrackFL"
  Integrator/1 -> Switch/1
  Gain/1 -> Integrator/1
  From Workspace/1 -> Switch/3
  Gain3/1 -> Surface Input Bus/4  "zTrackRR"
  Chirp Signal/1 -> Gain/1
  Surface Input Bus/1 -> Surface Model/1
  Gain1/1 -> Surface Input Bus/2  "zTrackFR"
  Gain2/1 -> Surface Input Bus/3  "zTrackRL"
  z_r_type/1 -> Switch/2

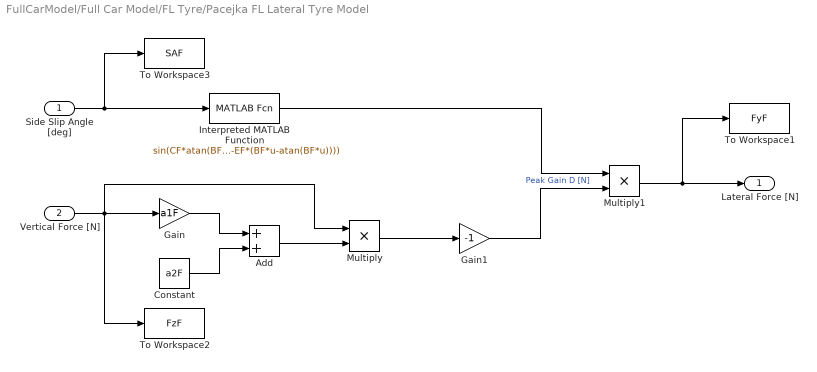
== system FullCarModel/Full Car Model/FL Tyre/Pacejka FL Lateral Tyre Model ==
  Side Slip Angle [deg] : Inport
  Vertical Force [N] : Inport  Port=2
  Add : Sum
  Constant : Constant  Value=a2F
  Gain : Gain  Gain=a1F
  Gain1 : Gain  Gain=-1
  Interpreted MATLAB Function : MATLABFcn  MATLABFcn=sin(CF*atan(BF*u-EF*(BF*u-atan(BF*u))))
  Multiply : Product
  Multiply1 : Product
  To Workspace1 : ToWorkspace  VariableName=FyF  SaveFormat=Timeseries  SampleTime=-1
  To Workspace2 : ToWorkspace  VariableName=FzF  SaveFormat=Timeseries  SampleTime=-1
  To Workspace3 : ToWorkspace  VariableName=SAF  SaveFormat=Timeseries  SampleTime=-1
  Lateral Force [N] : Outport  VectorParamsAs1DForOutWhenUnconnected=off
  wires:
  Vertical Force [N]/1 -> To Workspace2/1, Gain/1, Multiply/1
  Constant/1 -> Add/2
  Gain/1 -> Add/1
  Add/1 -> Multiply/2
  Multiply/1 -> Gain1/1
  Gain1/1 -> Multiply1/2  "Peak Gain D [N]"
  Side Slip Angle [deg]/1 -> To Workspace3/1, Interpreted MATLAB Function/1
  Interpreted MATLAB Function/1 -> Multiply1/1
  Multiply1/1 -> To Workspace1/1, Lateral Force [N]/1
